simulink model "math"  (Simulink 4.00)
settings: Solver=ode45  StartTime=0.0  StopTime=10.0  RelTol=1e-3
libraries: simulink3 x1
settings Model: LastModifiedBy=owner  LimitDataPoints=off  ExtModeTrigMode=oneshot  ExtModeArmWhenConnect=off

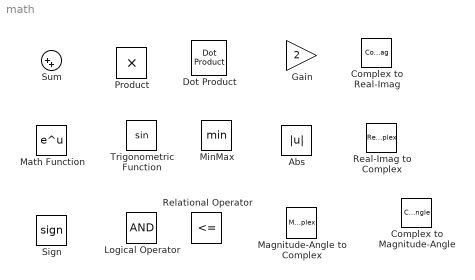
== system math ==
  Abs : Abs  SaturateOnIntegerOverflow=on
  Complex to Magnitude-Angle : ComplexToMagnitudeAngle  Output=MagnitudeAndAngle
  Complex to Real-Imag : ComplexToRealImag  Output=RealAndImag
  Dot Product : simulink3/Math/Dot Product
  Gain : Gain  Gain=2  Multiplication=Element-wise(K.*u)  SaturateOnIntegerOverflow=on
  Logical Operator : Logic  Operator=AND  Inputs=2
  Magnitude-Angle to Complex : MagnitudeAngleToComplex  Input=MagnitudeAndAngle  ConstantPart=0
  Math Function : Math  Operator=exp  OutputSignalType=auto
  MinMax : MinMax  Function=min  Inputs=1
  Product : Product  Inputs=2  Multiplication=Element-wise(.*)  SaturateOnIntegerOverflow=on
  Real-Imag to Complex : RealImagToComplex  Input=RealAndImag  ConstantPart=0
  Relational Operator : RelationalOperator  Operator=<=
  Sign : Signum
  Sum : Sum  Inputs=|++  SaturateOnIntegerOverflow=on
  Trigonometric Function : Trigonometry  Operator=sin  OutputSignalType=auto
  wires:
  ? -> Sum/2
